simulink model "LADRCsiso"  (R2022b)
settings: Solver=VariableStepAuto  StartTime=0.0  StopTime=10.0  RelTol=1e-3
values from neighbouring files (symbols this model uses):
  A = [0 1; 0 0]    [main.m]
  B = [b0; 0]    [main.m]
  b0 = K/T    (= 1)    [main.m]
  C = [1 0]    [main.m]
  K = 1    [main.m]
  Kp = 4/Tsettle    (= 4)    [main.m]
  L = [-2*S_eso; S_eso^2]    [main.m]
  T = 1    [main.m]
settings Model: Creator=d066566  LastModifiedBy=d066566

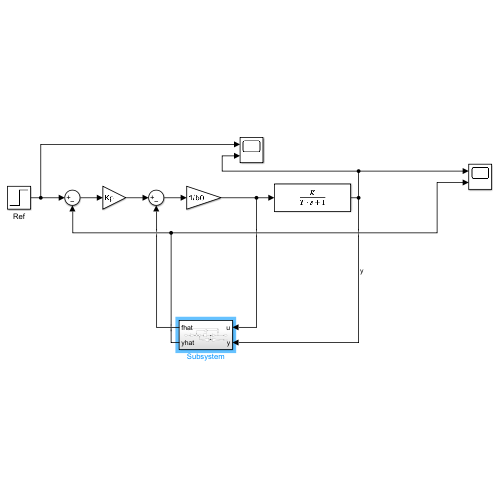
[thumbnail: Simulink's stored preview of the top-level diagram]
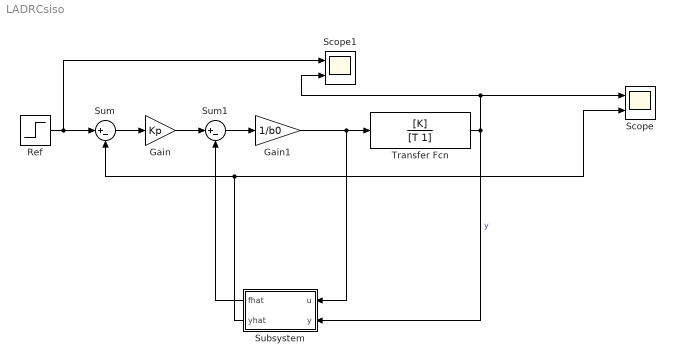
== system LADRCsiso ==
  Gain : Gain  Gain=Kp
  Gain1 : Gain  Gain=1/b0
  Ref : Step  SampleTime=0
  Scope : Scope  NumInputPorts=2
  Scope1 : Scope  NumInputPorts=2
  Subsystem : Subsystem
  Sum : Sum  Inputs=|+-
  Sum1 : Sum  Inputs=|+-
  Transfer Fcn : TransferFcn  Numerator=[K]  Denominator=[T 1]
  wires:
  Ref/1 -> Scope1/1, Sum/1
  Sum/1 -> Gain/1
  Gain/1 -> Sum1/1
  Sum1/1 -> Gain1/1
  Gain1/1 -> Subsystem/1(u), Transfer Fcn/1
  Transfer Fcn/1 -> Subsystem/2(y), Scope1/2, Scope/1  "y"
  Subsystem/2(yhat) -> Scope/2, Sum/2
  Subsystem/1(fhat) -> Sum1/2

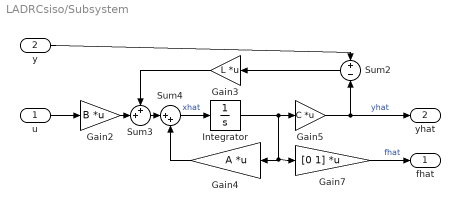
== system LADRCsiso/Subsystem ==
  u : Inport
  y : Inport  Port=2
  Gain2 : Gain  Gain=B  Multiplication=Matrix(K*u)
  Gain3 : Gain  Gain=L  Multiplication=Matrix(K*u)
  Gain4 : Gain  Gain=A  Multiplication=Matrix(K*u)
  Gain5 : Gain  Gain=C  Multiplication=Matrix(K*u)
  Gain7 : Gain  Gain=[0 1]  Multiplication=Matrix(K*u)
  Integrator : Integrator
  Sum2 : Sum  Inputs=+|-
  Sum3 : Sum  Inputs=++|
  Sum4 : Sum  Inputs=|++
  fhat : Outport
  yhat : Outport  Port=2
  wires:
  Gain3/1 -> Sum3/1
  Gain5/1 -> yhat/1, Sum2/2  "yhat"
  Gain2/1 -> Sum3/2
  Gain7/1 -> fhat/1  "fhat"
  Sum2/1 -> Gain3/1
  y/1 -> Sum2/1
  Sum3/1 -> Sum4/1
  u/1 -> Gain2/1
  Sum4/1 -> Integrator/1  "xhat"
  Gain4/1 -> Sum4/2
  Integrator/1 -> Gain5/1, Gain7/1, Gain4/1
